simulink model "KakmanFilterVoltageExample__Simtestbench"  (R2023b)
settings: Solver=FixedStepAuto  StartTime=0.0  StopTime=10.0  FixedStep=Ts  RelTol=1e-3
undefined symbols (not defined in the file): Discrete, Time, Ts
libraries: ctrlSharedLib x1
settings Model: Creator=leoni  LastModifiedBy=leoni

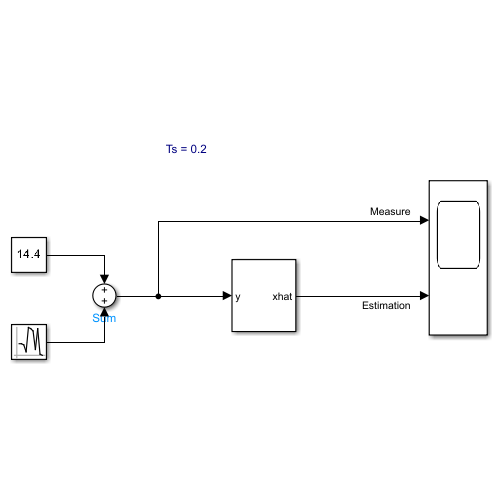
[thumbnail: Simulink's stored preview of the top-level diagram]
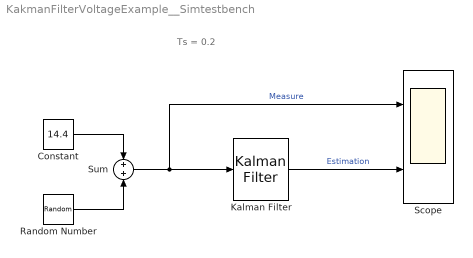
== system KakmanFilterVoltageExample__Simtestbench ==
  note: Ts = 0.2
  Constant : Constant  Value=14.4
  Kalman Filter : ctrlSharedLib/Kalman Filter  TimeDomain=Discrete-Time  UseCurrentEstimator=on  ModelSource=Individual A, B, C, D matrices  ModelSourceVariable=ss(0.95,1,1,0,1)  A=1  B=1  C=1  D=0  NumberOfStates=1  NumberOfInputs=1  NumberOfOutputs=1  InitialEstimateSource=Dialog  X0=14  P0=10  UseK=off  UseGH=off  NumberOfProcessNoiseInputs=1  G=1  TimeInvariantG=on  H=0  TimeInvariantH=on  Q=0.01  TimeInvariantQ=on  R=4  TimeInvariantR=on  N=0  TimeInvariantN=on  AddInputPort=off  AddEnablePort=off  OutputEstimatedY=off  OutputP=off  Ts=-1
  Random Number : RandomNumber  Variance=4  SampleTime=Ts
  Scope : Scope  NumInputPorts=2
  Sum : Sum  Inputs=+|+
  wires:
  Constant/1 -> Sum/1
  Random Number/1 -> Sum/2
  Sum/1 -> Scope/1, Kalman Filter/1  "Measure"
  Kalman Filter/1 -> Scope/2  "Estimation"
